simulink model "MotorCtrl_FOC_Math"  (R2025b)
settings: Solver=FixedStepDiscrete  StartTime=0.0  StopTime=5  FixedStep=MC_Sim_BaseStep  RelTol=1e-3  EnableMultiTasking=on
values from neighbouring files (symbols this model uses):
  MC_ADC_BitNum = 0.0    [MotorControlDataDictionary_Math.sldd]
  MC_ADC_Offset = 0.0    [MotorControlDataDictionary_Math.sldd]
  MC_ADC_VRef = 1.0    [MotorControlDataDictionary_Math.sldd]
  MC_CSA_Gain = 1.0    [MotorControlDataDictionary_Math.sldd]
  MC_MOS_DeadTime = 1.3E-6    [MotorControlDataDictionary_Math.sldd]
  MC_Motor_Mechinal_Damp = 1.0E-5    [MotorControlDataDictionary_Math.sldd]
  MC_Motor_Mechinal_Fric = 0.0    [MotorControlDataDictionary_Math.sldd]
  MC_Motor_Mechinal_Inertia = 0.0103    [MotorControlDataDictionary_Math.sldd]
  MC_Motor_Phi = 0.0059190254913385806    [MotorControlDataDictionary_Math.sldd]
  MC_Motor_Rotor_Pn = 4.0    [MotorControlDataDictionary_Math.sldd]
  MC_Motor_Stator_Ld = 5.6345E-5    [MotorControlDataDictionary_Math.sldd]
  MC_Motor_Stator_Lq = 5.6345E-5    [MotorControlDataDictionary_Math.sldd]
  MC_Motor_Stator_Rs = 0.0286    [MotorControlDataDictionary_Math.sldd]
  MC_Param_CurrentPI_Ki = 0.0089705790612839825    [MotorControlDataDictionary_Math.sldd]
  MC_Param_CurrentPI_Kp = 0.283220860906427    [MotorControlDataDictionary_Math.sldd]
  MC_Param_CurrentPI_UdInteMax = 7.794228634059948    [MotorControlDataDictionary_Math.sldd]
  MC_Param_CurrentPI_UdInteMin = -7.794228634059948    [MotorControlDataDictionary_Math.sldd]
  MC_Param_CurrentPI_UdMax = 7.794228634059948    [MotorControlDataDictionary_Math.sldd]
  MC_Param_CurrentPI_UdMin = -7.794228634059948    [MotorControlDataDictionary_Math.sldd]
  MC_Param_CurrentPI_UqInteMax = 7.794228634059948    [MotorControlDataDictionary_Math.sldd]
  MC_Param_CurrentPI_UqInteMin = -7.794228634059948    [MotorControlDataDictionary_Math.sldd]
  MC_Param_CurrentPI_UqMax = 7.794228634059948    [MotorControlDataDictionary_Math.sldd]
  MC_Param_CurrentPI_UqMin = -7.794228634059948    [MotorControlDataDictionary_Math.sldd]
  MC_Param_Flux_Gamma = 750000.0    [MotorControlDataDictionary_Math.sldd]
  MC_Param_Flux_Lalpha = 5.6345E-5    [MotorControlDataDictionary_Math.sldd]
  MC_Param_Flux_Lbeta = 5.6345E-5    [MotorControlDataDictionary_Math.sldd]
  MC_Param_Flux_Ralpha = 0.0286    [MotorControlDataDictionary_Math.sldd]
  MC_Param_Flux_Rbeta = 0.0286    [MotorControlDataDictionary_Math.sldd]
  MC_Param_Luen_BEMFalpha = -17747.803709290976    [MotorControlDataDictionary_Math.sldd]
  MC_Param_Luen_BEMFbeta = -17747.803709290976    [MotorControlDataDictionary_Math.sldd]
  MC_Param_Luen_BEMFErr = 10.0    [MotorControlDataDictionary_Math.sldd]
  MC_Param_Luen_Currentalpha = -507.58718608572195    [MotorControlDataDictionary_Math.sldd]
  MC_Param_Luen_Currentbeta = -507.58718608572195    [MotorControlDataDictionary_Math.sldd]
  MC_Param_Luen_CurrentErr = 400.0    [MotorControlDataDictionary_Math.sldd]
  MC_Param_Luen_PLL_Ki = 0.24634532585119037    [MotorControlDataDictionary_Math.sldd]
  MC_Param_Luen_PLL_Kp = 125.66370614359172    [MotorControlDataDictionary_Math.sldd]
  MC_Param_Luen_Voltagealpha = 17747.803709290976    [MotorControlDataDictionary_Math.sldd]
  MC_Param_Luen_Voltagebeta = 17747.803709290976    [MotorControlDataDictionary_Math.sldd]
  MC_Param_PhasetoReal = 500.0    [MotorControlDataDictionary_Math.sldd]
  MC_Param_SMO_CoffA = 0.968326559588251    [MotorControlDataDictionary_Math.sldd]
  MC_Param_SMO_CoffB = 1.1074629514597569    [MotorControlDataDictionary_Math.sldd]
  MC_Param_SpeedCtrl_IdMax = 60.0    [MotorControlDataDictionary_Math.sldd]
  MC_Param_SpeedCtrl_IdMin = -60.0    [MotorControlDataDictionary_Math.sldd]
  MC_Param_SpeedCtrl_IqMax = 60.0    [MotorControlDataDictionary_Math.sldd]
  MC_Param_SpeedCtrl_IqMin = -60.0    [MotorControlDataDictionary_Math.sldd]
  MC_Param_SpeedPI_Ki = 0.57157085739428382    [MotorControlDataDictionary_Math.sldd]
  MC_Param_SpeedPI_Kp = 9.1114109857344836    [MotorControlDataDictionary_Math.sldd]
  MC_Param_SpeedtoTheta = 6.24E-5    [MotorControlDataDictionary_Math.sldd]
  MC_Param_SVPWM_DutyMax = 0.98    [MotorControlDataDictionary_Math.sldd]
  MC_Param_SVPWM_DutyMin = 0.02    [MotorControlDataDictionary_Math.sldd]
  MC_Param_SVPWM_SampleOffset1 = 0.02    [MotorControlDataDictionary_Math.sldd]
  MC_Param_SVPWM_SampleOffset2 = 0.015    [MotorControlDataDictionary_Math.sldd]
  MC_Param_SVPWM_SampleValid = 0.0096153846153846159    [MotorControlDataDictionary_Math.sldd]
  MC_Param_Zero = 0.0    [MotorControlDataDictionary_Math.sldd]
  MC_Sample_CurrentNoise = 1.0E-15    [MotorControlDataDictionary_Math.sldd]
  MC_Sample_Rs = 0.002    [MotorControlDataDictionary_Math.sldd]
  MC_Sample_VbusNoise = 1.0E-15    [MotorControlDataDictionary_Math.sldd]
  MC_Sim_BaseStep = 2.08E-8    [MotorControlDataDictionary_Math.sldd]
  MC_Sim_HFTStep = 6.24E-5    [MotorControlDataDictionary_Math.sldd]
  MC_Sim_MFTStep = 0.0019968    [MotorControlDataDictionary_Math.sldd]
libraries: simulink x28, nesl_utility x19, fl_lib x14, ee_lib x13, autolibpmsminterior x2, autolibinverter x1
(part 3 of 8)

== system MotorCtrl_FOC_Math/HFTask/getCurrentPredict ==
  note: 开发日志：
      | 2025.03.26:
      | 1、完成两节拍的电流预测
      | 2025.03.27：
      | 1、采用延时2个周期的采样电流和延时1个周期的设定电压进行延时1个周期的电机电流预测
  Ud1 : Inport
  Id : Inport  Port=2
  Uq1 : Inport  Port=3
  Iq : Inport  Port=4
  Wm : Inport  Port=5
  Add : Sum  Inputs=+++
  Add1 : Sum  Inputs=++-
  Add2 : Sum
  Constant : Constant  Value=MC_Motor_Phi  OutDataTypeStr=single
  Gain1 : Gain  Gain=MC_Sim_HFTStep/MC_Motor_Stator_Lq
  Gain4 : Gain  Gain=MC_Sim_HFTStep/MC_Motor_Stator_Ld
  Gain5 : Gain  Gain=1-(MC_Sim_HFTStep*MC_Motor_Stator_Rs/MC_Motor_Stator_Ld)
  Gain6 : Gain  Gain=MC_Sim_HFTStep/MC_Motor_Stator_Lq
  Gain7 : Gain  Gain=1-(MC_Sim_HFTStep*MC_Motor_Stator_Rs/MC_Motor_Stator_Lq)
  Gain8 : Gain  Gain=MC_Sim_HFTStep*MC_Motor_Stator_Ld/MC_Motor_Stator_Lq
  Gain9 : Gain  Gain=(MC_Sim_HFTStep*MC_Motor_Stator_Lq/MC_Motor_Stator_Ld)
  Product : Product
  Product1 : Product
  Id_Pre : Outport
  Iq_Pre : Outport  Port=2
  wires:
  [Iq] -> Gain7/1
  [Wm] -> Product1/1
  Iq/1 -> [Iq]
  Gain4/1 -> Add/1  "Ud_Id1"
  [Iq] -> Gain9/1
  [Uq1] -> Gain6/1
  Gain9/1 -> Product/1
  Constant/1 -> Gain1/1
  Product/1 -> Add/3  "Iq_Id1"
  [Ud1] -> Gain4/1
  Gain6/1 -> Add1/1  "Uq_Iq1"
  Gain7/1 -> Add1/2  "Iq_Iq1"
  Gain5/1 -> Add/2  "Id_Id1"
  [Id] -> Gain8/1
  Product1/1 -> Add1/3  "Id_Iq1"
  Gain8/1 -> Add2/1
  [Wm] -> Product/2
  Id/1 -> [Id]
  Add2/1 -> Product1/2
  [Id] -> Gain5/1
  Wm/1 -> [Wm]
  Gain1/1 -> Add2/2
  Add/1 -> Id_Pre/1  "Id1"
  Add1/1 -> Iq_Pre/1  "Iq1"
  Ud1/1 -> [Ud1]
  Uq1/1 -> [Uq1]

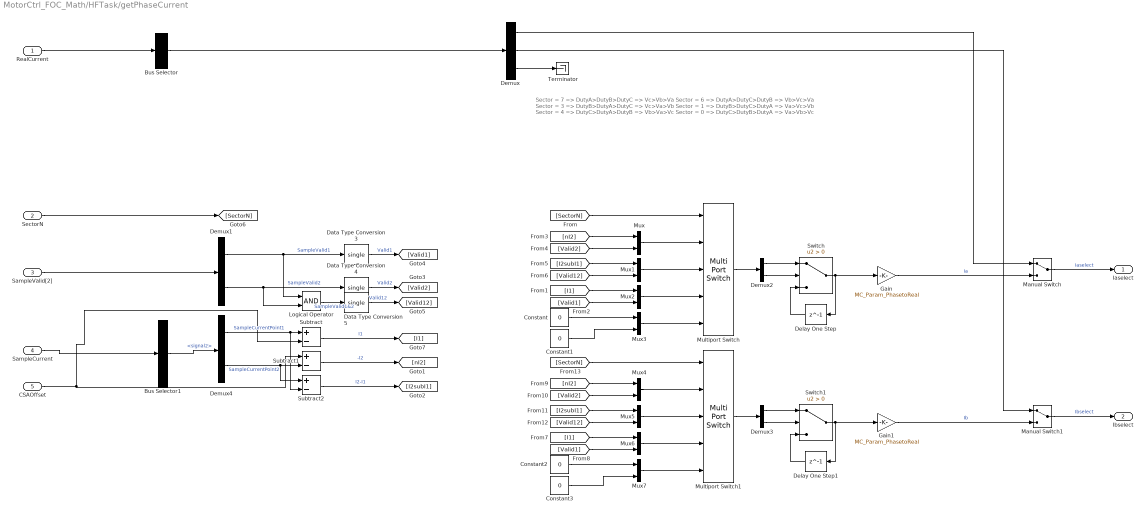
== system MotorCtrl_FOC_Math/HFTask/getPhaseCurrent ==
  note: Sector = 7 => DutyA>DutyB>DutyC => Vc>Vb>Va
      | Sector = 6 => DutyA>DutyC>DutyB => Vb>Vc>Va
      | Sector = 3 => DutyB>DutyA>DutyC => Vc>Va>Vb
      | Sector = 1 => DutyB>DutyC>DutyA => Va>Vc>Vb
      | Sector = 4 => DutyC>DutyA>DutyB => Vb>Va>Vc
      | Sector = 0 => DutyC>DutyB>DutyA => Va>Vb>Vc
  RealCurrent : Inport
  SectorN : Inport  Port=2
  SampleValid[2] : Inport  Port=3
  SampleCurrent : Inport  Port=4
  CSAOffset : Inport  Port=5
  Bus Selector : BusSelector  OutputSignals=PhaseI  OutputAsBus=on
  Bus Selector1 : BusSelector  OutputSignals=signal2
  Constant{,1..3} (4 alike) : Constant  Value=0  OutDataTypeStr=single
  Data Type Conversion3 : DataTypeConversion  OutDataTypeStr=single  RndMeth=Simplest  SaturateOnIntegerOverflow=off
  Data Type Conversion4 : DataTypeConversion  OutDataTypeStr=single  RndMeth=Simplest  SaturateOnIntegerOverflow=off
  Data Type Conversion5 : DataTypeConversion  OutDataTypeStr=single  RndMeth=Simplest  SaturateOnIntegerOverflow=off
  Delay One Step : Delay  DelayLength=1
  Delay One Step1 : Delay  DelayLength=1
  Demux : Demux  Outputs=3
  Demux{1..4} (4 alike) : Demux  Outputs=2
  Gain : Gain  Gain=MC_Param_PhasetoReal
  Gain1 : Gain  Gain=MC_Param_PhasetoReal
  Logical Operator : Logic  AllPortsSameDT=off  OutDataTypeStr=boolean
  Manual Switch : ManualSwitch
  Manual Switch1 : ManualSwitch
  Multiport Switch : MultiPortSwitch  DataPortOrder=Specify indices  DataPortIndices={[7,6],[3,4],[0,1]}  DataPortForDefault=Additional data port  SaturateOnIntegerOverflow=off  InputSameDT=off
  Multiport Switch1 : MultiPortSwitch  DataPortOrder=Specify indices  DataPortIndices={[3,1],[7,0],[6,4]}  DataPortForDefault=Additional data port  SaturateOnIntegerOverflow=off  InputSameDT=off
  Mux{,1..7} (8 alike) : Mux  Inputs=2
  Subtract : Sum  Inputs=+-
  Subtract1 : Sum  Inputs=+-
  Subtract2 : Sum  Inputs=+-
  Switch : Switch  Criteria=u2 > Threshold  SaturateOnIntegerOverflow=off  InputSameDT=off
  Switch1 : Switch  Criteria=u2 > Threshold  SaturateOnIntegerOverflow=off  InputSameDT=off
  Terminator : Terminator
  Iaselect : Outport
  Ibselect : Outport  Port=2
  wires:
  RealCurrent/1 -> Bus Selector/1
  Bus Selector/1 -> Demux/1
  Manual Switch/1 -> Iaselect/1  "Iaselect"
  Demux/3 -> Terminator/1
  Manual Switch1/1 -> Ibselect/1  "Ibselect"
  Multiport Switch1/1 -> Demux3/1
  Demux3/2 -> Switch1/2
  Demux3/1 -> Switch1/1
  Switch1/1 -> Delay One Step1/1, Gain1/1
  Delay One Step1/1 -> Switch1/3
  Gain1/1 -> Manual Switch1/2  "Ib"
  Gain/1 -> Manual Switch/2  "Ia"
  Delay One Step/1 -> Switch/3
  Switch/1 -> Gain/1, Delay One Step/1
  Demux2/1 -> Switch/1
  Demux2/2 -> Switch/2
  Multiport Switch/1 -> Demux2/1
  [SectorN] -> Multiport Switch1/1
  Mux4/1 -> Multiport Switch1/2
  Mux5/1 -> Multiport Switch1/3
  Mux6/1 -> Multiport Switch1/4
  [I1] -> Mux6/1
  [Valid1] -> Mux6/2
  [nI2] -> Mux4/1
  [Valid2] -> Mux4/2
  [Valid12] -> Mux5/2
  [I2subI1] -> Mux5/1
  Mux7/1 -> Multiport Switch1/5
  Constant2/1 -> Mux7/1
  Constant3/1 -> Mux7/2
  Subtract/1 -> [I1]  "I1"
  Subtract1/1 -> [nI2]  "-I2"
  Data Type Conversion5/1 -> [Valid12]  "Valid12"
  Data Type Conversion4/1 -> [Valid2]  "Valid2"
  Data Type Conversion3/1 -> [Valid1]  "Valid1"
  Subtract2/1 -> [I2subI1]  "I2-I1"
  Constant1/1 -> Mux3/2
  Constant/1 -> Mux3/1
  Mux3/1 -> Multiport Switch/5
  [I2subI1] -> Mux1/1
  [Valid12] -> Mux1/2
  [Valid2] -> Mux/2
  [nI2] -> Mux/1
  [Valid1] -> Mux2/2
  [I1] -> Mux2/1
  [SectorN] -> Multiport Switch/1
  SectorN/1 -> [SectorN]
  Mux2/1 -> Multiport Switch/4
  Mux1/1 -> Multiport Switch/3
  Mux/1 -> Multiport Switch/2
  Logical Operator/1 -> Data Type Conversion5/1  "SampleValid1&2"
  Demux1/2 -> Data Type Conversion4/1, Logical Operator/2  "SampleValid2"
  Demux1/1 -> Data Type Conversion3/1, Logical Operator/1  "SampleValid1"
  SampleValid[2]/1 -> Demux1/1
  Demux4/2 -> Subtract2/1, Subtract1/2  "SampleCurrentPoint2"
  CSAOffset/1 -> Subtract1/1, Subtract/2
  Demux4/1 -> Subtract2/2, Subtract/1  "SampleCurrentPoint1"
  Bus Selector1/1 -> Demux4/1  "<signal2>"
  SampleCurrent/1 -> Bus Selector1/1
  Demux/1 -> Manual Switch/1
  Demux/2 -> Manual Switch1/1

== system MotorCtrl_FOC_Math/HFTask/getSinCos ==
  Theta : Inport
  Sin : Trigonometry
  Sin1 : Trigonometry  Operator=cos
  SinTheta : Outport
  CosTheta : Outport  Port=2
  wires:
  Theta/1 -> Sin1/1, Sin/1
  Sin/1 -> SinTheta/1
  Sin1/1 -> CosTheta/1

== system MotorCtrl_FOC_Math/HFTask/invParkTransform ==
  Ud : Inport
  Uq : Inport  Port=2
  SinTheta : Inport  Port=3
  CosTheta : Inport  Port=4
  Add : Sum
  Product{,1..3} (4 alike) : Product
  Subtract : Sum  Inputs=+-
  Ualpha : Outport
  Ubeta : Outport  Port=2
  wires:
  Uq/1 -> Product3/1, Product1/1
  Subtract/1 -> Ualpha/1  "Ualpha"
  CosTheta/1 -> Product/2, Product3/2
  SinTheta/1 -> Product2/2, Product1/2
  Product/1 -> Subtract/1
  Product1/1 -> Subtract/2
  Ud/1 -> Product/1, Product2/1
  Product2/1 -> Add/1
  Product3/1 -> Add/2
  Add/1 -> Ubeta/1  "Ubeta"

== system MotorCtrl_FOC_Math/HFTask/karmalObservor ==
  In1 : Inport
  Out1 : Outport
  wires:
  In1/1 -> Out1/1

== system MotorCtrl_FOC_Math/HFTask/scvmobservor ==
  Vd : Inport
  Vq : Inport  Port=2
  Id : Inport  Port=3
  Iq : Inport  Port=4
  getW : Subsystem
  wires:
  Vd/1 -> getW/1(Vd)
  Vq/1 -> getW/2(Vq)
  Id/1 -> getW/3(Id)
  Iq/1 -> getW/4(Iq)

== system MotorCtrl_FOC_Math/HFTask/smo ==
  Valpha : Inport
  Vbeta : Inport  Port=2
  Ialpha : Inport  Port=3
  Ibeta : Inport  Port=4
  getE : Subsystem
  getSpeedandTheta : Subsystem
  Speed : Outport
  Theta : Outport  Port=2
  wires:
  Valpha/1 -> getE/1(Valpha)
  Vbeta/1 -> getE/2(Vbeta)
  Ialpha/1 -> getE/3(Ialpha)
  Ibeta/1 -> getE/4(Ibeta)
  getE/1(Ealpha) -> getSpeedandTheta/1(Ealpha)
  getE/2(Ebeta) -> getSpeedandTheta/2(Ebeta)
  getSpeedandTheta/1(Speed) -> Speed/1
  getSpeedandTheta/2(Theta) -> Theta/1

== system MotorCtrl_FOC_Math/HFTask/svpwm ==
  Valpha : Inport
  Vbeta : Inport  Port=2
  Vdc : Inport  Port=3
  Ia : Inport  Port=4
  Ib : Inport  Port=5
  PhaseShortEnableFlag : Inport  Port=6
  Terminator : Terminator
  getVoltageExchange : Subsystem
  setDTCompelte : Subsystem
  setPhaseandSample_ORS_Double : Subsystem
  DutySVPWM : Outport
  SamplePoint : Outport  Port=2
  SampleValid : Outport  Port=3
  SectorN : Outport  Port=4
  wires:
  Valpha/1 -> getVoltageExchange/1(Valpha)
  Vbeta/1 -> getVoltageExchange/2(Vbeta)
  Vdc/1 -> getVoltageExchange/3(Vdc)
  getVoltageExchange/1(Va) -> setDTCompelte/1(Va)
  getVoltageExchange/2(Vb) -> setDTCompelte/2(Vb)
  getVoltageExchange/3(Vc) -> setDTCompelte/3(Vc)
  getVoltageExchange/4(Vmed) -> setDTCompelte/4(Vmed)
  Ia/1 -> setDTCompelte/5(Ia)
  Ib/1 -> setDTCompelte/6(ib)
  setDTCompelte/1(SectorN) -> SectorN/1, setPhaseandSample_ORS_Double/1(SectorN)
  setDTCompelte/2(DutyLMS) -> setPhaseandSample_ORS_Double/2(DutyLMS)
  setPhaseandSample_ORS_Double/1(DutySVPWM) -> DutySVPWM/1
  setPhaseandSample_ORS_Double/2(SamplePoint) -> SamplePoint/1
  setPhaseandSample_ORS_Double/3(SampleValid) -> SampleValid/1
  PhaseShortEnableFlag/1 -> Terminator/1

== system MotorCtrl_FOC_Math/HFTask/voltageLimit ==
  UdRef : Inport
  UqRef : Inport  Port=2
  Umax : Inport  Port=3
  Add : Sum
  Compare To Constant : simulink/Logic and Bit Operations/Compare To Constant  relop=<=  const=0  OutDataTypeStr=boolean
  Compare To Constant1 : simulink/Logic and Bit Operations/Compare To Constant  relop=>=  const=0  OutDataTypeStr=boolean
  Constant : Constant  Value=0  OutDataTypeStr=single
  Gain : Gain  Gain=-1
  Gain1 : Gain  Gain=-1
  Product : Product
  Saturation Dynamic : simulink/Discontinuities/Saturation Dynamic  OutMin=[]  OutMax=[]  OutDataTypeStr=Inherit: Same as second input  OutDataType=fixdt(1, 16)  OutScaling=2^-10  DoSatur=off
  Sqrt : Sqrt
  Subtract : Sum  Inputs=+-
  Switch : Switch  Criteria=u2 > Threshold  SaturateOnIntegerOverflow=off  InputSameDT=off
  Switch1 : Switch  Criteria=u2 > Threshold  SaturateOnIntegerOverflow=off  InputSameDT=off
  Switch2 : Switch  Criteria=u2 > Threshold  SaturateOnIntegerOverflow=off  InputSameDT=off
  Ud : Outport
  Uq : Outport  Port=2
  wires:
  Add/1 -> Product/1
  Subtract/1 -> Product/2
  Product/1 -> Compare To Constant/1, Sqrt/1
  Compare To Constant/1 -> [UdOverFlow]
  Sqrt/1 -> Gain/1, Saturation Dynamic/1
  Gain/1 -> Saturation Dynamic/3
  UdRef/1 -> [UdRef]
  UqRef/1 -> [UqRef]
  Umax/1 -> [Umax]
  [Umax] -> Subtract/1, Add/1
  [UdRef] -> Add/2, Subtract/2
  [UqRef] -> Saturation Dynamic/2
  Saturation Dynamic/1 -> Switch/3
  [UdOverFlow] -> Switch/2
  Constant/1 -> Switch/1
  Switch/1 -> Uq/1  "UqLimit"
  Switch1/1 -> Ud/1  "UdLimit"
  Switch2/1 -> Switch1/1
  [UdRef] -> Compare To Constant1/1
  Compare To Constant1/1 -> Switch2/2
  [Umax] -> Gain1/1, Switch2/1
  Gain1/1 -> Switch2/3
  [UdOverFlow] -> Switch1/2
  [UdRef] -> Switch1/3

== system MotorCtrl_FOC_Math/Hardware_Math/AngleProcess ==
  In1 : Inport
  Constant : Constant  Value=2*pi  SampleTime=-1
  Data Type Conversion : DataTypeConversion  OutDataTypeStr=single  SaturateOnIntegerOverflow=off  RndMeth=Floor
  Mod : Math  Operator=mod
  Out1 : Outport
  wires:
  Mod/1 -> Data Type Conversion/1
  In1/1 -> Mod/1
  Constant/1 -> Mod/2
  Data Type Conversion/1 -> Out1/1  "ThetaM"

== system MotorCtrl_FOC_Math/Hardware_Math/MotorHardware ==
  mec : Inport
  PWM : Inport  Port=2
  Bus Creator : BusCreator  Inputs=3
  Electrical Reference : fl_lib/Electrical/Electrical Elements/Electrical Reference
  Interior PMSM : autolibpmsminterior/Interior PMSM  port_config=Torque  sim_type=Discrete  Ts=MC_Sim_BaseStep  P=MC_Motor_Rotor_Pn  Rs=MC_Motor_Stator_Rs  Ldq=[MC_Motor_Stator_Ld MC_Motor_Stator_Lq]  KConstText=Permanent flux linkage constant (lambda_pm):  lambda_pm=MC_Motor_Phi  Ke=159.9771  mechanical=[MC_Motor_Mechinal_Inertia,MC_Motor_Mechinal_Damp,MC_Motor_Mechinal_Fric]  idq0=[0 0]  theta_init=0  omega_init=0  KConst=0.2205  lambda_pm_calc=0.2205  Kt=0.07  RefBlkName='autolibpmsminterior/Interior PMSM'  aMode=5
      settings: LibrarySourceBlock=mcblib/Electrical Systems/Motors/Interior PMSM
  InverterSim : Subsystem
      settings: PortSchema="{\"entries\":[{\"content\":{\"sides\":[{\"content\":{\"connectorIds\":[\"In1\",\"LConn1\",\"LConn2\",\"LConn3\"]},\"type\":\"ConnectorPlacement.EquallySpacedRectSide\",\"uuid\":\"2e5f838d-5170-43e4-b1ea-9f326f7142e0\"},{\"content\":{\"connectorIds\":[\"RConn1\",\"RConn2\",\"RConn3\",\"RConn4\",\"Out1\"],\"side\":\"RIGHT\"},\"type\":\"ConnectorPlacement.EquallySpacedRectSide\",\"uuid\":\"45e0921e-af98-47db-a55b-1ba25f6efcf4\"},{\"content\":{\"side\":\"TOP\"},\"type\":\"ConnectorPlacement.EquallySpacedRectSide\",\"uuid\":\"e2c729c4-40af-4664-b83b-786ffce64e92\"}]},\"type\":\"ConnectorPlacement.EquallySpacedConnector\",\"uuid\":\"1d5b8e8e-96ab-46b4-8630-102f3e39175a\"}],\"packageUris\":[\"http://schema.mathworks.com/mf0/Connector/R2020b\"],\"version\":\"1.0\"}"
  MotorMachineSim : Subsystem
  PMSM : ee_lib/Electromechanical/Permanent Magnet/PMSM  port_option=ee.enum.threePhasePort.expanded  winding_type=ee.enum.electromech.statorconfiguration.delta  machine_param=ee.enum.pmsm.parameterization.constant  nPolePairs=MC_Motor_Rotor_Pn  pmflux_param=ee.enum.pmflux.fluxlinkage  pm_flux_linkage=MC_Motor_Phi Wb  torque_constant=0.18 N*m/A  back_emf_constant=0.18 V*s/rad  stator_param=ee.enum.statorparam.LdLqL0  Ld=MC_Motor_Stator_Ld H  Lq=MC_Motor_Stator_Ld H  idVec=[-200, 0, 200] A  iqVec=[-200, 0, 200] A  LdMatrix=0.0002 * ones(3, 3) H  LqMatrix=0.0002 * ones(3, 3) H  PmMatrix=0.1 * ones(3, 3) Wb  ktMatrix=0.18 * ones(3, 3) N*m/A  keMatrix=0.18 * ones(3, 3) V*s/rad  L0=MC_Motor_Stator_L0 H  Ls=0.0002 H  Lm=-0.00002 H  Ms=0.00002 H  Rs=MC_Motor_Stator_Rs Ohm  zero_sequence=ee.enum.park.zerosequence.include  axes_param=ee.enum.rotorangle.daxis  loss_param=ee.enum.ironloss.none  losses_oc=[0, 0, 0] W  losses_sc=[0, 0, 0] W  f_losses=60 Hz  Isc_losses=95 A  J=MC_Motor_Mechinal_Inertia kg*m^2  lam=MC_Motor_Mechinal_Damp N*m*s/rad  i_d_specify=off  i_d_priority=None  i_d=0 A  i_d_nominal_specify=off  i_d_nominal_value=1  i_d_nominal_unit=A  i_q_specify=off  i_q_priority=None  i_q=0 A  i_q_nominal_specify=off  i_q_nominal_value=1  i_q_nominal_unit=A  torque_specify=off  torque_priority=None  torque=0 N*m  torque_nominal_specify=off  torque_nominal_value=1  torque_nominal_unit=N*m  angular_velocity_specify=off  angular_velocity_priority=High  angular_velocity=0 rpm  angular_velocity_nominal_specify=off  angular_velocity_nominal_value=1  angular_velocity_nominal_unit=rpm  angular_position_specify=off  angular_position_priority=High  angular_position=0 deg  angular_position_nominal_specify=off  angular_position_nominal_value=1  angular_position_nominal_unit=deg  alpha=3.93e-3 1/K  alpha_flux=-0.001 1/K  Tmeas=298.15 K  stator_thermal_mass=100 J/K  rotor_thermal_mass=200 J/K  Rm_percent_rotor=90  Rd_percent_rotor=30  temperatureA_specify=off  temperatureA_priority=High  temperatureA=25 degC  temperatureA_nominal_specify=off  temperatureA_nominal_value=1  temperatureA_nominal_unit=degC  temperatureB_specify=off  temperatureB_priority=High  temperatureB=25 degC  temperatureB_nominal_specify=off  temperatureB_nominal_value=1  temperatureB_nominal_unit=degC  temperatureC_specify=off  temperatureC_priority=High  temperatureC=25 degC  temperatureC_nominal_specify=off  temperatureC_nominal_value=1  temperatureC_nominal_unit=degC  temperatureR_specify=off  temperatureR_priority=High  temperatureR=25 degC  temperatureR_nominal_specify=off  temperatureR_nominal_value=1  temperatureR_nominal_unit=degC
      settings: InternalSimscapePortConfiguration="{\"Bottom\":[],\"Left\":[{\"id\":\"a\",\"label\":\"a\",\"type\":\"foundation.electrical.electrical\"},{\"id\":\"b\",\"label\":\"b\",\"type\":\"foundation.electrical.electrical\"},{\"id\":\"c\",\"label\":\"c\",\"type\":\"foundation.electrical.electrical\"}],\"Right\":[{\"id\":\"R\",\"label\":\"R\",\"type\":\"foundation.mechanical.rotational.rotational\"},{\"id\":\"C\",\"label\":\"C\",\"type\":\"foundation.mechanical.rotational.rotational\"}],\"Top\":[]}"
  PS-Simulink Converter : nesl_utility/PS-Simulink Converter  PhysicalDomain=network_engine_domain  SubClassName=ps_output  LeftPortType=input  RightPortType=output  PseudoPeriodic=off  Frequencies=[]  VectorFormat=inherit  Unit=inherit  AffineConversion=off
  PhaseMeasureSim : Subsystem
  Voltage Sensor : fl_lib/Electrical/Electrical Sensors/Voltage Sensor
  Voltage Source : ee_lib/Sources/Voltage Source  dc_voltage=0 V  ac_voltage=0 V  ac_shift=0 rad  ac_frequency=60 Hz  noise_mode=ee.enum.sources.noise.Disabled  PSD=0 V^2/Hz  sample_time=1e-3 s  repeatability=ee.enum.sources.repeatability.NotRepeatable  user_seed=0  auto_seed=3890346746  i_specify=off  i_priority=None  i=0 A  i_nominal_specify=off  i_nominal_value=1  i_nominal_unit=A  v_specify=off  v_priority=None  v=0 V  v_nominal_specify=off  v_nominal_value=1  v_nominal_unit=V
  Vabc : Outport
  Iabc : Outport  Port=2
  m : Outport  Port=3
  Vbus : Outport  Port=4
  Current : Outport  Port=5
  wires:
  [Vbus] -> Vbus/1  "Vbus"
  InverterSim/1(Ibuss) -> Current/1  "Ibuss"
  PS-Simulink Converter/1 -> [Vbus]
  PWM/1 -> InverterSim/1(Drive)
  mec/1 -> MotorMachineSim/1(LoadTorque)
  PhaseMeasureSim/1(Vabc) -> Vabc/1
  PhaseMeasureSim/2(Iabc) -> Iabc/1
  MotorMachineSim/1(Torque_M) -> Bus Creator/1  "Te"
  MotorMachineSim/2(W_M) -> Bus Creator/2  "Wm"
  MotorMachineSim/3(Angle_M) -> Bus Creator/3  "ThetaM"
  Bus Creator/1 -> m/1
  ? -> Interior PMSM/1
  Interior PMSM/1 -> ?
  Interior PMSM/2 -> ?
  Interior PMSM/3 -> ?
  ? -> Interior PMSM/2
  connections:
  Voltage Source/LConn1 -- InverterSim/LConn1 -- Voltage Sensor/LConn1
  Electrical Reference/LConn1 -- InverterSim/LConn2 -- InverterSim/LConn3 -- Voltage Sensor/RConn2 -- Voltage Source/RConn1
  Voltage Sensor/RConn1 -- PS-Simulink Converter/LConn1
  MotorMachineSim/LConn1 -- PMSM/RConn1
  PMSM/RConn2 -- MotorMachineSim/LConn2
  PhaseMeasureSim/RConn1 -- PMSM/LConn1
  PhaseMeasureSim/RConn2 -- PMSM/LConn2
  PhaseMeasureSim/RConn3 -- PMSM/LConn3
  InverterSim/RConn4 -- PhaseMeasureSim/LConn4
  InverterSim/RConn3 -- PhaseMeasureSim/LConn3
  InverterSim/RConn2 -- PhaseMeasureSim/LConn2
  InverterSim/RConn1 -- PhaseMeasureSim/LConn1

== system MotorCtrl_FOC_Math/Hardware_Math/PWMGenerate ==
  DutyABC : Inport
  SamplePoint : Inport  Port=2
  Compare To Constant : simulink/Logic and Bit Operations/Compare To Constant  relop=<=  const=1  OutDataTypeStr=boolean
  Data Type Conversion{,1,3..6} (6 alike) : DataTypeConversion  SaturateOnIntegerOverflow=off  RndMeth=Floor
  Data Type Conversion2 : DataTypeConversion  OutDataTypeStr=double  SaturateOnIntegerOverflow=off  RndMeth=Floor
  DeadTimeGenerate : Subsystem
  Mux : Mux  Inputs=6
  Rate Transition : RateTransition  OutPortSampleTime=MC_Sim_BaseStep
  Rate Transition1 : RateTransition  OutPortSampleTime=MC_Sim_BaseStep
  Relational Operator{,2..3,5} (4 alike) : RelationalOperator  OutDataTypeStr=boolean  RndMeth=Simplest  InputSameDT=off
  Relational Operator1 : RelationalOperator  Operator=<=  OutDataTypeStr=boolean  RndMeth=Simplest  InputSameDT=off
  Relational Operator4 : RelationalOperator  Operator=<=  OutDataTypeStr=boolean  RndMeth=Simplest  InputSameDT=off
  Relational Operator6 : RelationalOperator  Operator=<=  OutDataTypeStr=boolean  RndMeth=Simplest  InputSameDT=off
  Repeating Sequence : simulink/Sources/Repeating Sequence  rep_seq_t=[0 MC_Sim_HFTStep/2 MC_Sim_HFTStep]  rep_seq_y=[0 1 2]
  Repeating Sequence1 : simulink/Sources/Repeating Sequence  rep_seq_t=[0 MC_Sim_HFTStep/2 MC_Sim_HFTStep]  rep_seq_y=[2 1 0]
  Switch : Switch  Criteria=u2 > Threshold  SaturateOnIntegerOverflow=off  InputSameDT=off
  Gate : Outport
  CurrentSamplTrigger : Outport  Port=2
  wires:
  Data Type Conversion6/1 -> Mux/6  "PWMCDOWN"
  Data Type Conversion5/1 -> Mux/5  "PWMCUP"
  Data Type Conversion4/1 -> Mux/4  "PWMBDOWN"
  Data Type Conversion3/1 -> Mux/3  "PWMBUP"
  Data Type Conversion1/1 -> Mux/2  "PWMADOWN"
  Data Type Conversion/1 -> Mux/1  "PWMAUP"
  DeadTimeGenerate/6(GateCL) -> Relational Operator6/2
  DeadTimeGenerate/5(GateCH) -> Relational Operator5/2
  DeadTimeGenerate/4(GateBL) -> Relational Operator4/2
  DeadTimeGenerate/3(GateBH) -> Relational Operator2/2
  Relational Operator6/1 -> Data Type Conversion6/1
  Relational Operator5/1 -> Data Type Conversion5/1
  Relational Operator4/1 -> Data Type Conversion4/1
  Relational Operator2/1 -> Data Type Conversion3/1
  Relational Operator1/1 -> Data Type Conversion1/1
  Relational Operator/1 -> Data Type Conversion/1
  Repeating Sequence/1 -> Switch/1, Compare To Constant/1
  Repeating Sequence1/1 -> Switch/3
  DutyABC/1 -> DeadTimeGenerate/2(DutyABC)
  DeadTimeGenerate/1(GateAH) -> Relational Operator/2
  Switch/1 -> Rate Transition/1
  DeadTimeGenerate/2(GateAL) -> Relational Operator1/2
  Relational Operator3/1 -> Data Type Conversion2/1
  SamplePoint/1 -> Relational Operator3/2
  Data Type Conversion2/1 -> CurrentSamplTrigger/1  "CurrentSamplTrigger"
  Compare To Constant/1 -> Rate Transition1/1
  Mux/1 -> Gate/1  "Gate"
  Rate Transition/1 -> Relational Operator/1, Relational Operator1/1, Relational Operator3/1, Relational Operator6/1, Relational Operator5/1, Relational Operator4/1, Relational Operator2/1
  Rate Transition1/1 -> DeadTimeGenerate/1(FLag), Switch/2

== system MotorCtrl_FOC_Math/Hardware_Math/VbusSample ==
  Vbus : Inport
  ADCOffset : Constant  Value=0  SampleTime=-1
  ADCQuality : Gain
  Add : Sum
  Data Type Conversion3 : DataTypeConversion  OutDataTypeStr=single  SaturateOnIntegerOverflow=off  RndMeth=Floor
  VbusSample : Outport
  wires:
  Vbus/1 -> Add/2
  Add/1 -> ADCQuality/1
  ADCQuality/1 -> Data Type Conversion3/1
  ADCOffset/1 -> Add/1
  Data Type Conversion3/1 -> VbusSample/1  "PhaseI"

== system MotorCtrl_FOC_Math/Hardware_Math/currentSample ==
  SampleTrigger : Inport
  Current : Inport  Port=2
  getCurrentSample_ORS_Double : Subsystem  VariantControl=MC_Sample_Model==1 && MC_Sample_ORSType == 2
  getCurrentSample_ORS_Single : Subsystem  VariantControl=MC_Sample_Model==1 && MC_Sample_ORSType == 1
  getCurrentSample_TRS(Three) : Subsystem  VariantControl=MC_Sample_Model==3
  getCurrentSample_TRS(Two) : Subsystem  VariantControl=MC_Sample_Model==2
  SampleCurrent : Outport

== system MotorCtrl_FOC_Math/Hardware_Sim/AngleProcess ==
  In1 : Inport
  Constant : Constant  Value=2*pi  SampleTime=-1
  Mod : Math  Operator=mod
  Out1 : Outport
  wires:
  In1/1 -> Mod/1
  Constant/1 -> Mod/2
  Mod/1 -> Out1/1

== system MotorCtrl_FOC_Math/Hardware_Sim/PWMGenerate ==
  DutyABC : Inport
  SamplePoint : Inport  Port=2
  Compare To Constant : simulink/Logic and Bit Operations/Compare To Constant  relop=<=  const=1  OutDataTypeStr=boolean
  Data Type Conversion{,1,3..6} (6 alike) : DataTypeConversion  SaturateOnIntegerOverflow=off  RndMeth=Floor
  Data Type Conversion2 : DataTypeConversion  OutDataTypeStr=double  SaturateOnIntegerOverflow=off  RndMeth=Floor
  DeadTimeGenerate : Subsystem
  Mux : Mux  Inputs=3
  Rate Transition : RateTransition  OutPortSampleTime=MC_Sim_BaseStep
  Rate Transition1 : RateTransition  OutPortSampleTime=MC_Sim_BaseStep
  Relational Operator{,2..3,5} (4 alike) : RelationalOperator  OutDataTypeStr=boolean  RndMeth=Simplest  InputSameDT=off
  Relational Operator1 : RelationalOperator  Operator=<=  OutDataTypeStr=boolean  RndMeth=Simplest  InputSameDT=off
  Relational Operator4 : RelationalOperator  Operator=<=  OutDataTypeStr=boolean  RndMeth=Simplest  InputSameDT=off
  Relational Operator6 : RelationalOperator  Operator=<=  OutDataTypeStr=boolean  RndMeth=Simplest  InputSameDT=off
  Repeating Sequence : simulink/Sources/Repeating Sequence  rep_seq_t=[0 MC_Sim_HFTStep/2 MC_Sim_HFTStep]  rep_seq_y=[0 1 2]
  Repeating Sequence1 : simulink/Sources/Repeating Sequence  rep_seq_t=[0 MC_Sim_HFTStep/2 MC_Sim_HFTStep]  rep_seq_y=[2 1 0]
  Switch : Switch  Criteria=u2 > Threshold  SaturateOnIntegerOverflow=off  InputSameDT=off
  Terminator : Terminator
  Terminator1 : Terminator
  Terminator2 : Terminator
  Gate : Outport
  CurrentSamplTrigger : Outport  Port=2
  wires:
  Data Type Conversion5/1 -> Mux/3  "PWMCUP"
  Data Type Conversion3/1 -> Mux/2  "PWMBUP"
  Data Type Conversion/1 -> Mux/1  "PWMAUP"
  DeadTimeGenerate/6(GateCL) -> Relational Operator6/2
  DeadTimeGenerate/5(GateCH) -> Relational Operator5/2
  DeadTimeGenerate/4(GateBL) -> Relational Operator4/2
  DeadTimeGenerate/3(GateBH) -> Relational Operator2/2
  Relational Operator6/1 -> Data Type Conversion6/1
  Relational Operator5/1 -> Data Type Conversion5/1
  Relational Operator4/1 -> Data Type Conversion4/1
  Relational Operator2/1 -> Data Type Conversion3/1
  Relational Operator1/1 -> Data Type Conversion1/1
  Relational Operator/1 -> Data Type Conversion/1
  Repeating Sequence/1 -> Switch/1, Compare To Constant/1
  Repeating Sequence1/1 -> Switch/3
  DutyABC/1 -> DeadTimeGenerate/2(DutyABC)
  DeadTimeGenerate/1(GateAH) -> Relational Operator/2
  Switch/1 -> Rate Transition/1
  DeadTimeGenerate/2(GateAL) -> Relational Operator1/2
  Relational Operator3/1 -> Data Type Conversion2/1
  SamplePoint/1 -> Relational Operator3/2
  Data Type Conversion2/1 -> CurrentSamplTrigger/1  "CurrentSamplTrigger"
  Compare To Constant/1 -> Rate Transition1/1
  Mux/1 -> Gate/1  "Gate"
  Rate Transition/1 -> Relational Operator/1, Relational Operator1/1, Relational Operator3/1, Relational Operator6/1, Relational Operator5/1, Relational Operator4/1, Relational Operator2/1
  Rate Transition1/1 -> DeadTimeGenerate/1(FLag), Switch/2
  Data Type Conversion6/1 -> Terminator/1  "PWMCDOWN"
  Data Type Conversion4/1 -> Terminator1/1  "PWMBDOWN"
  Data Type Conversion1/1 -> Terminator2/1  "PWMADOWN"

== system MotorCtrl_FOC_Math/Hardware_Sim/VbusSample ==
  Vbus : Inport
  ADCOffset : Constant  Value=0  SampleTime=-1
  ADCQuality : Gain
  Add : Sum
  Data Type Conversion3 : DataTypeConversion  OutDataTypeStr=single  SaturateOnIntegerOverflow=off  RndMeth=Floor
  VbusSample : Outport
  wires:
  Vbus/1 -> Add/2
  Add/1 -> ADCQuality/1
  ADCQuality/1 -> Data Type Conversion3/1
  ADCOffset/1 -> Add/1
  Data Type Conversion3/1 -> VbusSample/1  "PhaseI"

== system MotorCtrl_FOC_Math/Hardware_Sim/currentSample ==
  SampleTrigger : Inport
  Current : Inport  Port=2
  getCurrentSample_ORS_Double : Subsystem  VariantControl=MC_Sample_Model==1 && MC_Sample_ORSType == 2
  getCurrentSample_ORS_Single : Subsystem  VariantControl=MC_Sample_Model==1 && MC_Sample_ORSType == 1
  getCurrentSample_TRS(Three) : Subsystem  VariantControl=MC_Sample_Model==3
  getCurrentSample_TRS(Two) : Subsystem  VariantControl=MC_Sample_Model==2
  SampleCurrent : Outport
